simulink model "DCmotor_block_simple"  (R2014b)
settings: Solver=ode45  StartTime=0.0  StopTime=10.0  RelTol=1e-3
values from neighbouring files (symbols this model uses):
  Asimple = -((kE*kM)/(J*R)+Cv)    [create_ss.m]
  Bsimple = kM/(J*R)    [create_ss.m]
settings Model: Creator=davidebo  LastModifiedBy=davidebo

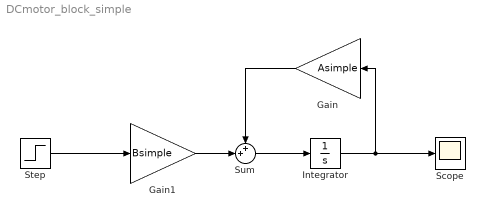
== system DCmotor_block_simple ==
  Gain : Gain  Gain=Asimple
  Gain1 : Gain  Gain=Bsimple
  Integrator : Integrator
  Scope : Scope
  Step : Step  After=24  SampleTime=0
  Sum : Sum  Inputs=++|
  wires:
  Integrator/1 -> Scope/1, Gain/1
  Sum/1 -> Integrator/1
  Gain/1 -> Sum/1
  Gain1/1 -> Sum/2
  Step/1 -> Gain1/1
